simulink model "pendulum_openloop_anim"  (Simulink 9.2)
settings: Solver=ode45  StartTime=0.0  StopTime=3  RelTol=1e-3  EnableMultiTasking=on
values from neighbouring files (symbols this model uses):
  g = 9.81    [pendulum_sys_init_NOsolution.m]    (also in pendulum_sys_init_WIP.m)
  kc = 2    [pendulum_sys_init_NOsolution.m]    (also in pendulum_sys_init_WIP.m)
  ke = 2    [pendulum_sys_init_NOsolution.m]    (also in pendulum_sys_init_WIP.m)
  l = 1    [pendulum_sys_init_NOsolution.m]    (also in pendulum_sys_init_WIP.m)
  M = 10    [pendulum_sys_init_NOsolution.m]    (also in pendulum_sys_init_WIP.m)
  m = 2    [pendulum_sys_init_NOsolution.m]    (also in pendulum_sys_init_WIP.m)
  ra = 10    [pendulum_sys_init_NOsolution.m]    (also in pendulum_sys_init_WIP.m)
  rr = .1    (= 0.1)    [pendulum_sys_init_NOsolution.m]    (also in pendulum_sys_init_WIP.m)
undefined symbols (not defined in the file or in its folder): pendolo_sys_diff
libraries: simulink x1, vrlib x1
settings Model: Creator=Titano  LastModifiedBy=Varazslav
settings OptimizationCC: BlockReduction=off  DefaultParameterBehavior=Inlined  BufferReuse=off  ExpressionDepthLimit=2147483647  InitFltsAndDblsToZero=on
settings DebuggingCC: SolverPrmCheckMsg=warning
settings SimscapeCC: SimscapeNormalizeSystem=off
settings SimMechanicsCC: VisDuringSimulation=on
settings ConfigurationSet: Description=SimMechanics 2G

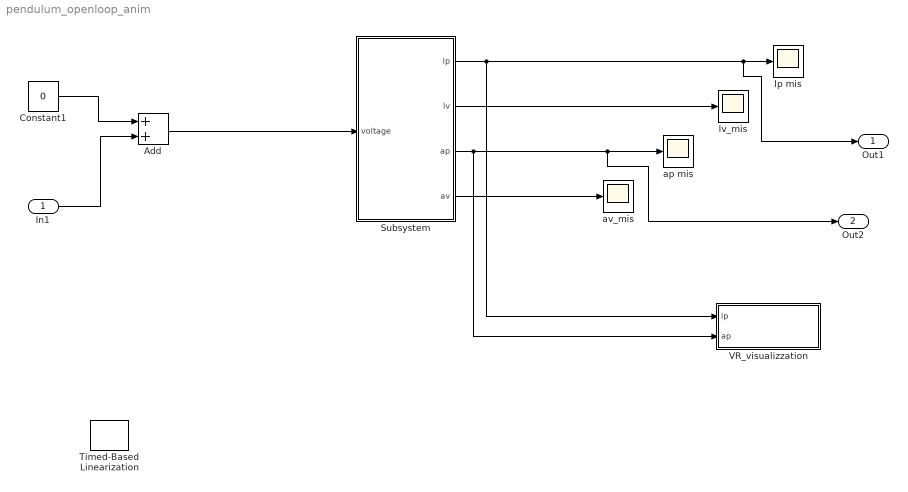
== system pendulum_openloop_anim ==
  In1 : Inport
  Add : Sum
  Constant1 : Constant  Value=0
  Subsystem : Subsystem
  Timed-Based Linearization : simulink/Model-Wide Utilities/Timed-Based Linearization  LinearizationTime=1  SampleTime=0
      settings: SourceProductName=Simulink  SourceProductBaseCode=SL
  VR_visualizzation : Subsystem
  ap mis : Scope
  "av_mis " : Scope
  lp mis : Scope
  lv_mis : Scope
  Out1 : Outport
  Out2 : Outport  Port=2
  wires:
  Subsystem/3(ap) -> VR_visualizzation/2(ap), Out2/1, ap mis/1
  In1/1 -> Add/2
  Constant1/1 -> Add/1
  Add/1 -> Subsystem/1(voltage)
  Subsystem/1(lp) -> VR_visualizzation/1(lp), Out1/1, lp mis/1
  Subsystem/2(lv) -> lv_mis/1
  Subsystem/4(av) -> "av_mis "/1

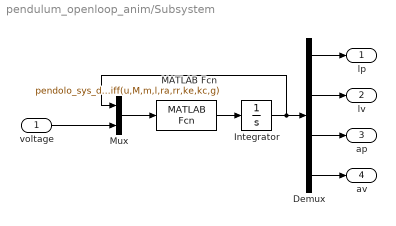
== system pendulum_openloop_anim/Subsystem ==
  voltage : Inport
  Demux : Demux
  Integrator : Integrator  InitialCondition=[0 0.0 0 0]
  MATLAB Fcn : MATLABFcn  MATLABFcn=pendolo_sys_diff(u,M,m,l,ra,rr,ke,kc,g)
  Mux : Mux  Inputs=2
  lp : Outport
  lv : Outport  Port=2
  ap : Outport  Port=3
  av : Outport  Port=4
  wires:
  MATLAB Fcn/1 -> Integrator/1
  Integrator/1 -> Demux/1, Mux/1
  Demux/4 -> av/1
  Demux/3 -> ap/1
  Demux/2 -> lv/1
  Demux/1 -> lp/1
  Mux/1 -> MATLAB Fcn/1
  voltage/1 -> Mux/2

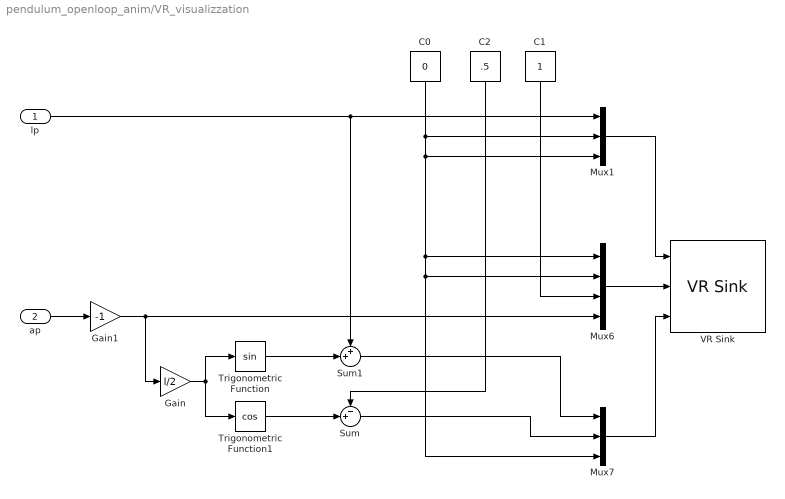
== system pendulum_openloop_anim/VR_visualizzation ==
  lp : Inport
  ap : Inport  Port=2
  C0 : Constant  Value=0
  C1 : Constant
  C2 : Constant  Value=.5
  Gain : Gain  Gain=l/2
  Gain1 : Gain  Gain=-1
  Mux1 : Mux  Inputs=3
  Mux6 : Mux
  Mux7 : Mux  Inputs=3
  Sum : Sum  Inputs=-+|
  Sum1 : Sum  Inputs=++|
  Trigonometric Function : Trigonometry
  Trigonometric Function1 : Trigonometry  Operator=cos
  VR Sink : vrlib/VR Sink  InstantiateOnLoad=on  SampleTime=0.02  ViewEnable=on  RemoteChange=off  RemoteView=off  FieldsWritten=carrello.translation.3.1.double#asta.rotation.4.1.double#asta.translation.3.1.double  WorldFileName=vrml1.wrl  AutoView=on  VideoDimensions=[]  AllowVariableSize=off  FigureProperties="{'Position', 'Name', 'Viewpoint', 'CameraBound', 'CameraDirection', 'CameraPosition', 'CameraUpVector', 'ZoomFactor', 'Antialiasing', 'Headlight', 'Lighting', 'NavPanel', 'Sound', 'StatusBar', 'Stereo3D', 'Stereo3DCameraOffset', 'Stereo3DHIT', 'ToolBar', 'Textures', 'Transparency', 'Triad', 'Wireframe', 'NavZones', 'NavMode', 'NavSpeed', 'CaptureFileFormat', 'CaptureFileName', 'Record2DCompressMethod', 'Record2DCompressQuality', 'Record2D', 'Record2DFileName', 'Record2DFPS'; [6.2566666666666663e+02   1.7633333333333337e+02   5.7599999999999989e+02   4.2000000000000000e+02], '', '', 'on', [3.4694469519536142e-17   0.0000000000000000e+00  -1.0000000000000000e+00], [8.5056186752640062e-01   0.0000000000000000e+00   4.9887710779360424e+00], [0.0000000000000000e+00   1.0000000000000000e+00   0.0000000000000000e+00], [1.0000000000000000e+00], 'on', 'on', 'on', 'halfbar', 'on', 'on', 'off', [1.0000000149011612e-01], [0.0000000000000000e+00], 'on', 'on', 'on', 'none', 'off', 'off', 'walk', 'normal', 'tif', '%f_anim_%n.tif', 'auto', [7.5000000000000000e+01], 'off', '%f_anim_%n.avi', [1.5000000000000000e+01]}"
      settings: SourceProductBaseCode=VR
  wires:
  Mux1/1 -> VR Sink/1
  Mux6/1 -> VR Sink/2
  Mux7/1 -> VR Sink/3
  lp/1 -> Mux1/1, Sum1/1
  C0/1 -> Mux1/2, Mux1/3, Mux6/1, Mux6/2, Mux7/3
  ap/1 -> Gain1/1
  C1/1 -> Mux6/3
  Trigonometric Function/1 -> Sum1/2
  Trigonometric Function1/1 -> Sum/2
  Sum1/1 -> Mux7/1
  Sum/1 -> Mux7/2
  C2/1 -> Sum/1
  Gain/1 -> Trigonometric Function/1, Trigonometric Function1/1
  Gain1/1 -> Mux6/4, Gain/1
